simulink model "sampleModel1672"  (R2023a)
settings: Solver=VariableStepAuto  StartTime=0.0  StopTime=10.0  RelTol=1e-3
libraries: hdlsllib x4, simulink x1
settings Model: Creator=user1  LastModifiedBy=user1

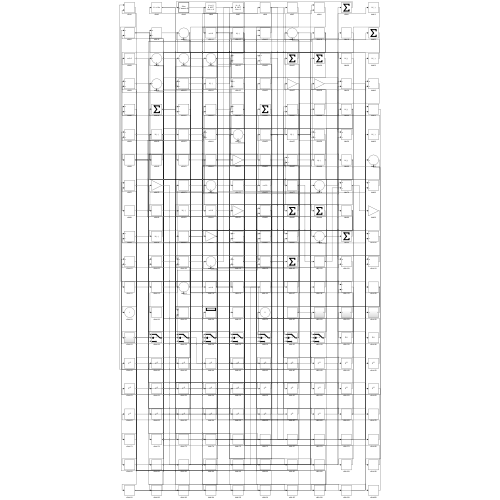
[thumbnail: Simulink's stored preview of the top-level diagram]
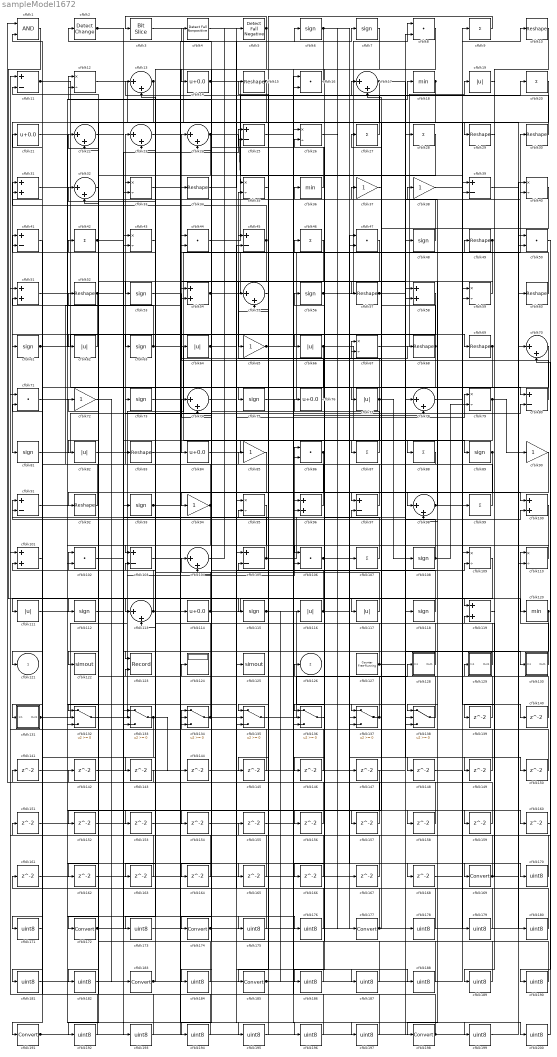
== system sampleModel1672 ==
  cfblk1 : Logic  AllPortsSameDT=off  OutDataTypeStr=boolean
  cfblk{10,15,29..30,34,49,52,57,60,68..69,83,92} (13 alike) : Reshape
  cfblk{31,51,54,58,96,100..101,119} (8 alike) : Sum
  cfblk{8,16,44,47,50,71,86,102,106} (9 alike) : DotProduct  OutDataTypeStr=Inherit: Inherit via internal rule
  cfblk{11,25,39,41,45,80,91,97,103,105} (10 alike) : Sum  Inputs=+-
  cfblk{13,17,22..24,32,55,70,74,78,98,104,113} (13 alike) : Sum  Inputs=|++
  cfblk{9,20,27..28,42,46,87..88,99,107} (10 alike) : Sum  Inputs=+
  cfblk{6..7,48,53,56,61,63,73,75,81,89,93,108,112,115,118} (16 alike) : Signum
  cfblk{12,26,33,35,40,43,59,67,79,95,109..110} (12 alike) : Product  Inputs=*/  RndMeth=Zero  SaturateOnIntegerOverflow=on
  cfblk{19,62,64,66,77,82,111,116..117} (9 alike) : Abs  SaturateOnIntegerOverflow=off
  cfblk{14,21,76,84,114} (5 alike) : Bias  Bias=0.0  SaturateOnIntegerOverflow=off
  cfblk120 : MinMax
  cfblk122 : ToWorkspace  VariableName=simout  SaveFormat=Timeseries  SampleTime=-1
  cfblk123 : Record  FileSettingsInternal="{\"entries\":[{\"content\":{\"excelSettings\":{\"content\":{},\"type\":\"Streamout.ExcelSettings\"}},\"type\":\"Streamout.FileSettingStorage\",\"uuid\":\"\"}],\"packageUris\":[\"http:\\/\\/schema.mathworks.com\\/mf0\\/streamout_blocks\\/R2020a\"],\"version\":\"1.0\"}"  Layout=[1 1]  SignalsInternal="{\"entries\":[{\"content\":{},\"type\":\"RecordBlkView.InputSignals\",\"uuid\":\"\"}],\"packageUris\":[\"http:\\/\\/schema.mathworks.com\\/mf0\\/streamout_blocks\\/R2020a\"],\"version\":\"1.0\"}"  VisualizationBindings="{\"xyplotplugin\":{\"info\":[{\"series\":[{\"bindingParametersList\":[{\"parameter\":\"X-Axis\",\"signalID\":2749,\"signalName\":\"cfblk89\"},{\"parameter\":\"Y-Axis\",\"signalID\":2753,\"signalName\":\"cfblk183\"}],\"seriesID\":25889}],\"subplotID\":1}]}}"  CompatibilityTag=XY  st=-1
  cfblk124 : Display
  cfblk125 : ToWorkspace  VariableName=simout  SaveFormat=Timeseries  SampleTime=-1
  cfblk127 : hdlsllib/Sources/Counter Free-Running  NumBits=16  tsamp=-1
  cfblk128 : Subsystem
      settings: LibrarySourceBlock=|
      | hdlsllib/Ports &
      | Subsystems/Subsystem
  cfblk129 : Subsystem
      settings: LibrarySourceBlock=|
      | hdlsllib/Ports &
      | Subsystems/Subsystem
  cfblk130 : Subsystem
      settings: LibrarySourceBlock=|
      | hdlsllib/Ports &
      | Subsystems/Subsystem
  cfblk131 : Subsystem
      settings: LibrarySourceBlock=|
      | hdlsllib/Ports &
      | Subsystems/Subsystem
  cfblk{132..138} (7 alike) : Switch  SaturateOnIntegerOverflow=off  InputSameDT=off
  cfblk{139..168} (30 alike) : Delay  SampleTime=1
  cfblk{169,172,174,177,183,185,191,198} (8 alike) : DataTypeConversion  SaturateOnIntegerOverflow=off  RndMeth=Floor
  cfblk{170..171,173,175..176,178..182,184,186..190,192..197,199..200} (24 alike) : DataTypeConversion  OutDataTypeStr=uint8  SaturateOnIntegerOverflow=off  RndMeth=Floor
  cfblk18 : MinMax
  cfblk2 : simulink/Logic and Bit Operations/Detect Change  vinit=0  OutDataTypeStr=boolean
      settings: LibrarySourceBlock=|
      | hdlsllib/Logic and Bit
      | Operations/Detect
      | Change
  cfblk3 : hdlsllib/Logic and Bit Operations/Bit Slice  lidx=7  ridx=0
  cfblk36 : MinMax
  cfblk{37..38,65,72,85,90,94} (7 alike) : Gain
  cfblk4 : hdlsllib/Logic and Bit Operations/Detect Fall Nonpositive  vinit=0  OutDataTypeStr=boolean
  cfblk5 : hdlsllib/Logic and Bit Operations/Detect Fall Negative  vinit=0  OutDataTypeStr=boolean
  cfblk121 : Outport  VectorParamsAs1DForOutWhenUnconnected=off
  cfblk126 : Outport  Port=2  VectorParamsAs1DForOutWhenUnconnected=off
  wires:
  cfblk104/1 -> cfblk5/1
  cfblk56/1 -> cfblk8/1, cfblk138/2, cfblk107/1, cfblk168/1
  cfblk37/1 -> cfblk97/1
  cfblk79/1 -> cfblk90/1, cfblk166/1
  cfblk84/1 -> cfblk88/1
  cfblk93/1 -> cfblk97/2, cfblk195/1
  cfblk9/1 -> cfblk75/1
  cfblk17/1 -> cfblk81/1, cfblk150/1
  cfblk1/1 -> cfblk112/1
  cfblk67/1 -> cfblk19/1
  cfblk36/1 -> cfblk2/1
  cfblk52/1 -> cfblk132/3, cfblk158/1
  cfblk92/1 -> cfblk24/1
  cfblk72/1 -> cfblk183/1
  cfblk28/1 -> cfblk172/1
  cfblk44/1 -> cfblk20/1
  cfblk53/1 -> cfblk84/1
  cfblk131/1(Out1) -> cfblk86/1, cfblk165/1
  cfblk130/1(Out1) -> cfblk110/1
  cfblk94/1 -> cfblk23/1, cfblk173/1
  cfblk129/1(Out1) -> cfblk27/1
  cfblk31/1 -> cfblk80/1
  cfblk24/1 -> cfblk35/1, cfblk43/2
  cfblk118/1 -> cfblk73/1
  cfblk66/1 -> cfblk89/1, cfblk102/2
  cfblk5/1 -> cfblk3/1, cfblk23/2
  cfblk132/1 -> cfblk46/1
  cfblk14/1 -> cfblk99/1, cfblk160/1
  cfblk59/1 -> cfblk57/1
  cfblk45/1 -> cfblk92/1, cfblk31/1
  cfblk136/1 -> cfblk36/1
  cfblk58/1 -> cfblk132/1
  cfblk76/1 -> cfblk35/2
  cfblk54/1 -> cfblk49/1, cfblk187/1
  cfblk42/1 -> cfblk25/1, cfblk197/1
  cfblk26/1 -> cfblk177/1
  cfblk4/1 -> cfblk87/1
  cfblk35/1 -> cfblk135/1
  cfblk98/1 -> cfblk38/1, cfblk140/1
  cfblk88/1 -> cfblk86/2
  cfblk15/1 -> cfblk63/1, cfblk54/2, cfblk152/1, cfblk153/1
  cfblk119/1 -> cfblk134/1
  cfblk3/1 -> cfblk110/2
  cfblk75/1 -> cfblk30/1
  cfblk47/1 -> cfblk113/1
  cfblk77/1 -> cfblk45/1, cfblk133/2, cfblk136/3, cfblk108/1
  cfblk51/1 -> cfblk114/1
  cfblk38/1 -> cfblk10/1
  cfblk80/1 -> cfblk54/1
  cfblk63/1 -> cfblk125/1, cfblk41/2
  cfblk62/1 -> cfblk61/1
  cfblk12/1 -> cfblk59/1
  cfblk91/1 -> cfblk135/2
  cfblk60/1 -> cfblk44/1
  cfblk46/1 -> cfblk122/1
  cfblk61/1 -> cfblk69/1, cfblk18/1, cfblk115/1, cfblk176/1
  cfblk43/1 -> cfblk103/1
  cfblk30/1 -> cfblk13/1
  cfblk135/1 -> cfblk128/1(In1)
  cfblk95/1 -> cfblk174/1
  cfblk11/1 -> cfblk77/1, cfblk109/1
  cfblk83/1 -> cfblk44/2
  cfblk116/1 -> cfblk34/1, cfblk106/2, cfblk149/1
  cfblk101/1 -> cfblk191/1
  cfblk73/1 -> cfblk68/1
  cfblk107/1 -> cfblk76/1
  cfblk115/1 -> cfblk137/1, cfblk78/2
  cfblk117/1 -> cfblk104/1
  cfblk120/1 -> cfblk133/3, cfblk143/1
  cfblk20/1 -> cfblk136/1
  cfblk127/1 -> cfblk91/1, cfblk100/2
  cfblk113/1 -> cfblk6/1, cfblk31/2
  cfblk97/1 -> cfblk42/1
  cfblk32/1 -> cfblk62/1
  cfblk34/1 -> cfblk7/1
  cfblk65/1 -> cfblk100/1, cfblk145/1
  cfblk16/1 -> cfblk14/1
  cfblk105/1 -> cfblk78/1, cfblk52/1
  cfblk87/1 -> cfblk12/1
  cfblk86/1 -> cfblk104/2, cfblk163/1, cfblk186/1
  cfblk106/1 -> cfblk147/1, cfblk148/1
  cfblk27/1 -> cfblk17/1
  cfblk18/1 -> cfblk53/1, cfblk117/1, cfblk164/1
  cfblk10/1 -> cfblk29/1
  cfblk78/1 -> cfblk9/1
  cfblk112/1 -> cfblk96/2
  cfblk114/1 -> cfblk33/1, cfblk120/1, cfblk111/1, cfblk109/2
  cfblk55/1 -> cfblk185/1
  cfblk69/1 -> cfblk137/3, cfblk162/1
  cfblk96/1 -> cfblk4/1
  cfblk70/1 -> cfblk198/1
  cfblk89/1 -> cfblk138/1, cfblk123/1, cfblk182/1
  cfblk49/1 -> cfblk65/1, cfblk98/2
  cfblk23/1 -> cfblk98/1
  cfblk134/1 -> cfblk32/1, cfblk79/1
  cfblk133/1 -> cfblk144/1, cfblk171/1
  cfblk22/1 -> cfblk93/1
  cfblk110/1 -> cfblk106/1
  cfblk103/1 -> cfblk67/1
  cfblk48/1 -> cfblk11/2
  cfblk137/1 -> cfblk22/1, cfblk102/1
  cfblk68/1 -> cfblk37/1, cfblk131/1(In1)
  cfblk138/1 -> cfblk126/1
  cfblk100/1 -> cfblk132/2
  cfblk33/1 -> cfblk58/2
  cfblk99/1 -> cfblk51/2
  cfblk128/1(Out1) -> cfblk41/1
  cfblk2/1 -> cfblk135/3, cfblk154/1
  cfblk6/1 -> cfblk119/1, cfblk134/2, cfblk136/2, cfblk167/1
  cfblk81/1 -> cfblk80/2
  cfblk8/1 -> cfblk94/1
  cfblk13/1 -> cfblk33/2, cfblk82/1
  cfblk41/1 -> cfblk121/1
  cfblk64/1 -> cfblk66/1, cfblk156/1
  cfblk71/1 -> cfblk169/1
  cfblk108/1 -> cfblk91/2, cfblk79/2
  cfblk57/1 -> cfblk48/1, cfblk130/1(In1), cfblk40/2
  cfblk29/1 -> cfblk139/1
  cfblk139/1 -> cfblk96/1
  cfblk140/1 -> cfblk67/2
  cfblk141/1 -> cfblk137/2
  cfblk142/1 -> cfblk22/2
  cfblk143/1 -> cfblk1/1
  cfblk144/1 -> cfblk8/2
  cfblk145/1 -> cfblk13/2
  cfblk7/1 -> cfblk146/1
  cfblk146/1 -> cfblk51/1
  cfblk149/1 -> cfblk32/2
  cfblk150/1 -> cfblk119/2
  cfblk151/1 -> cfblk134/3
  cfblk152/1 -> cfblk133/1
  cfblk153/1 -> cfblk16/2
  cfblk50/1 -> cfblk155/1
  cfblk156/1 -> cfblk25/2
  cfblk40/1 -> cfblk157/1
  cfblk157/1 -> cfblk105/1
  cfblk158/1 -> cfblk11/1
  cfblk111/1 -> cfblk159/1
  cfblk159/1 -> cfblk113/2
  cfblk161/1 -> cfblk47/2
  cfblk162/1 -> cfblk45/2
  cfblk163/1 -> cfblk1/2
  cfblk164/1 -> cfblk103/2
  cfblk165/1 -> cfblk43/1
  cfblk166/1 -> cfblk12/2
  cfblk167/1 -> cfblk24/2
  cfblk168/1 -> cfblk59/2
  cfblk169/1 -> cfblk50/1, cfblk129/1(In1), cfblk105/2
  cfblk155/1 -> cfblk170/1
  cfblk170/1 -> cfblk71/1
  cfblk171/1 -> cfblk71/2
  cfblk172/1 -> cfblk83/1, cfblk47/1
  cfblk173/1 -> cfblk28/1
  cfblk174/1 -> cfblk50/2, cfblk60/1
  cfblk102/1 -> cfblk175/1
  cfblk175/1 -> cfblk95/1
  cfblk176/1 -> cfblk95/2
  cfblk177/1 -> cfblk151/1, cfblk17/2, cfblk124/1
  cfblk178/1 -> cfblk26/1
  cfblk148/1 -> cfblk179/1
  cfblk179/1 -> cfblk26/2
  cfblk39/1 -> cfblk180/1
  cfblk180/1 -> cfblk15/1
  cfblk109/1 -> cfblk181/1
  cfblk181/1 -> cfblk39/1
  cfblk182/1 -> cfblk39/2
  cfblk183/1 -> cfblk123/2, cfblk118/1, cfblk58/1
  cfblk90/1 -> cfblk184/1
  cfblk184/1 -> cfblk72/1
  cfblk185/1 -> cfblk138/3, cfblk116/1
  cfblk186/1 -> cfblk55/1
  cfblk187/1 -> cfblk55/2
  cfblk74/1 -> cfblk188/1
  cfblk188/1 -> cfblk56/1
  cfblk19/1 -> cfblk189/1
  cfblk189/1 -> cfblk74/1
  cfblk160/1 -> cfblk190/1
  cfblk190/1 -> cfblk74/2
  cfblk191/1 -> cfblk178/1, cfblk40/1, cfblk64/1
  cfblk147/1 -> cfblk192/1
  cfblk192/1 -> cfblk101/1
  cfblk82/1 -> cfblk193/1
  cfblk193/1 -> cfblk101/2
  cfblk85/1 -> cfblk194/1
  cfblk194/1 -> cfblk141/1
  cfblk195/1 -> cfblk85/1
  cfblk21/1 -> cfblk196/1
  cfblk196/1 -> cfblk142/1
  cfblk197/1 -> cfblk21/1
  cfblk198/1 -> cfblk161/1, cfblk16/1
  cfblk25/1 -> cfblk199/1
  cfblk199/1 -> cfblk70/1
  cfblk154/1 -> cfblk200/1
  cfblk200/1 -> cfblk70/2

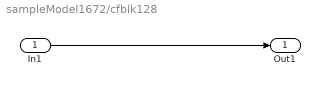
== system sampleModel1672/cfblk128 ==
  In1 : Inport
  Out1 : Outport
  wires:
  In1/1 -> Out1/1

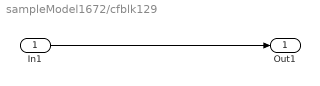
== system sampleModel1672/cfblk129 ==
  In1 : Inport
  Out1 : Outport
  wires:
  In1/1 -> Out1/1

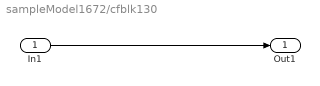
== system sampleModel1672/cfblk130 ==
  In1 : Inport
  Out1 : Outport
  wires:
  In1/1 -> Out1/1

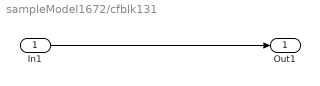
== system sampleModel1672/cfblk131 ==
  In1 : Inport
  Out1 : Outport
  wires:
  In1/1 -> Out1/1
